simulink library "M160_lib"  (Simulink 7.8)
settings: Solver=FixedStepDiscrete  StartTime=0.0  StopTime=10.0  RelTol=1e-3
PreLoadFcn:
  | update_path
undefined symbols (not defined in the file): Afr_atCool2facLambdaReqCorr_CUR_x, Afr_atCool2facLambdaReqCorr_CUR_y, Afr_atMani2facLambdaReqCorr_CUR_x, Afr_atMani2facLambdaReqCorr_CUR_y, Afr_facLambdaReqMan, Afr_facRatioMan, Afr_facStoich, Afr_flgLambdaReqOverride, Afr_flgRatioOverride, Afr_rpmEngSpdfacRelAir2facLambdaReqBase_MAP_x, Afr_rpmEngSpdfacRelAir2facLambdaReqBase_MAP_y, Afr_rpmEngSpdfacRelAir2facLambdaReqBase_MAP_z, Ais_flgAirInjReacPumpOverride, Ais_stAirInjReacPumpMan, Amc_flgAirMassFlowOverride, Amc_uSens2AirMassFlow_CUR_x, Amc_uSens2AirMassFlow_CUR_y, Amc_uSensMaxValid, Amc_uSensMinValid, Amf_facRelAirMan, Amf_flgAirMassPerStrOverride, Amf_flgRelAirOverride, Amf_flgSwitch2AirMassFlowMeter, Amf_mAirPerStrMan, Amf_pManiEngSpd2facRelAirCorr_MAP_x, Amf_pManiEngSpd2facRelAirCorr_MAP_y, Amf_pManiEngSpd2facRelAirCorr_MAP_z, Amf_rpmEngSpd2facTempCorr_CUR_x, Amf_rpmEngSpd2facTempCorr_CUR_y, Amf_shcSpecGasConst_C, Amf_volEngDisp_C, Apv_facAirPumpRateMan, Apv_factor, Apv_flgAirPumpRateOverride, Apv_tiPeriod_C, Bvc_rVoltDivHigh, Bvc_rVoltDivLow, Bvc_uBattMax, Bvc_uBattMin, CDRV_E_OK_, Cov_facChOverVlvRateMan, Cov_factor, Cov_flgChOverVlvRateOverride, Cov_tiPeriod_C, Cpc_atManiTmp2facPresCorr_CUR_x, Cpc_atManiTmp2facPresCorr_CUR_y, Cpc_flgPChargeOverride, Cpc_uSens2pManiBase_CUR_x, Cpc_uSens2pManiBase_CUR_y, Ctc_rPullUp_C, Ctc_rSens2atCool_CUR_x, Ctc_rSens2atCool_CUR_y, Ctc_uSensMaxValid, Ctc_uSensMinValid, Ctc_uSupply, Doh_OutputDiagnosisOverride, dummy_facAirPumpRateReq, dummy_facChOverVlvRateReq, dummy_flgInterCoolerOverride, dummy_flgKl50Override ... (+243)
libraries: simulink x36, ehooks_lib x3
(part 1 of 8)
CloseFcn:
  | clear
settings Model: Creator=WLB9FE  LastModifiedBy=Tiger

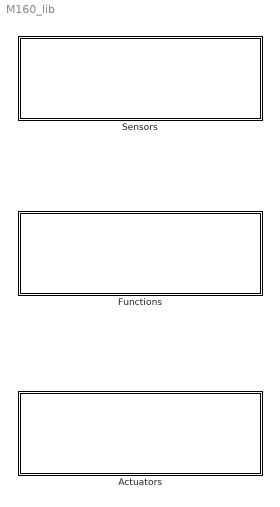
== system M160_lib ==
  Actuators : Subsystem
      mask Display: fprintf('actuators')
  Functions : Subsystem
      mask Display: fprintf('functions')
  Sensors : Subsystem
      mask Display: fprintf('sensors')

== system M160_lib/Actuators ==
  Ais : Subsystem
      mask Type: Actuators
      mask Description: AirInjectionReactorPump
      mask Display:
      | image(imread('AirInjectionReactorPump.jpg'))
      | port_label('input',1,'Opm_idxMode')
      | port_label('input',2,'dummy_stAirInjReacPump')
      | port_label('output',1,'Ais_stDiagnosis')
      | port_label('output',2,'Ais_flgError')
  Apv : Subsystem
      mask Type: Actuators
      mask Description: AirPumpValve
      mask Display:
      | image(imread('AirPumpValve.jpg'))
      | port_label('input',1,'Opm_idxMode')
      | port_label('input',2,'dummy_facAirPumpRate')
      | port_label('output',1,'Apv_stDiagnosis')
      | port_label('output',2,'Apv_flgError')
  Cov : Subsystem
      mask Type: Actuators
      mask Description: ChangeOverValve
      mask Display:
      | image(imread('ChangeOverValve.jpg'))
      | port_label('input',1,'Opm_idxMode')
      | port_label('input',2,'dummy_facChOverVlvRate')
      | port_label('output',1,'Cov_stDiagnosis')
      | port_label('output',2,'Cov_flgError')
  Fps : Subsystem
      mask Type: Actuators
      mask Description: FuelPump
      mask Display:
      | image(imread('FuelPump.jpg'))
      | port_label('input',1,'Opm_idxMode')
      | port_label('input',2,'dummy_stFuelPump')
      | port_label('output',1,'Fps_stDiagnosis')
      | port_label('output',2,'Fps_flgError')
  Icc : Subsystem
      mask Type: Actuators
      mask Description: IgnitionCoil
      mask Display:
      | image(imread('IgnitionCoil.jpg'))
      | port_label('input',1,'Opm_idxMode')
      | port_label('input',2,'Iac_flgIgnCutoff')
      | port_label('input',3,'Iac_degIgnIdleSpeed')
      | port_label('output',1,'Icc_flgError')
  Ics : Subsystem
      mask Type: Actuators
      mask Description: Intercooler
      mask Display:
      | image(imread('Intercooler.jpg'))
      | port_label('input',1,'Opm_idxMode')
      | port_label('input',2,'dummy_stIntercooler')
      | port_label('output',1,'Ics_stDiagnosis')
      | port_label('output',2,'Ics_flgError')
  Ivc : Subsystem
      mask Type: Actuators
      mask Description: InjectionValve
      mask Display:
      | image(imread('InjectionValve.jpg'))
      | port_label('input',1,'Opm_idxMode')
      | port_label('input',2,'Itc_flgInjCutoff')
      | port_label('input',3,'Itc_tiInj')
      | port_label('input',4,'Itc_tiBattDelay')
      | port_label('output',1,'Ivc_flgError')
  Mrs : Subsystem
      mask Type: Actuators
      mask Description: MainRelais
      mask Display:
      | image(imread('MainRelais.jpg'))
      | port_label('input',1,'Opm_idxMode')
      | port_label('input',2,'dummy_stMainRelais')
      | port_label('output',1,'Mrs_stDiagnosis')
      | port_label('output',2,'Mrs_flgError')
  Str : Subsystem
      mask Type: Actuators
      mask Description: Starter
      mask Display:
      | image(imread('Starter.jpg'))
      | port_label('input',1,'Opm_idxMode')
      | port_label('input',2,'Stc_stStarter')
      | port_label('output',1,'Str_stDiagnosis')
      | port_label('output',2,'Str_flgError')
  Tvc : Subsystem
      mask Type: Actuators
      mask Description: ThrottleValve
      mask Display:
      | image(imread('ThrottleValve.jpg'))
      | port_label('input',1,'Opm_idxMode')
      | port_label('input',2,'dummy_facThrValveReq')
      | port_label('output',1,'Tvc_stDiagnosis')
      | port_label('output',2,'Tvc_flgError')
  Wcs : Subsystem
      mask Type: Actuators
      mask Description: WaterCooler
      mask Display:
      | image(imread('WaterCooler.jpg'))
      | port_label('input',1,'Opm_idxMode')
      | port_label('input',2,'Ctc_atCool')
      | port_label('output',1,'Wcs_stDiagnosis')
      | port_label('output',2,'Wcs_flgError')
  Wgc : Subsystem
      mask Type: Actuators
      mask Description: WasteGate
      mask Display:
      | image(imread('WasteGate.jpg'))
      | port_label('input',1,'Opm_idxMode')
      | port_label('input',2,'T2t_facWasteGateRate')
      | port_label('output',1,'Wgc_stDiagnosis')
      | port_label('output',2,'Wgc_flgError')

== system M160_lib/Functions ==
  Afr : Subsystem
      mask Type: Functions
      mask Description: AirFuelRatio
      mask Display:
      | image(imread('AirFuelRatio.jpg'))
      | port_label('input',1,'Epm_rpmEngSpd')
      | port_label('input',2,'Mtc_atMani')
      | port_label('input',3,'Ctc_atCool')
      | port_label('input',4,'Amf_facRelAir')
      | port_label('output',1,'Afr_facLambdaReq')
      | port_label('output',2,'Afr_facRatio')
  Amf : Subsystem
      mask Type: Functions
      mask Description: AirMassFlow
      mask Display:
      | image(imread('AirMassFlow.jpg'))
      | port_label('input',1,'Epm_rpmEngSpd')
      | port_label('input',2,'Mtc_atMani')
      | port_label('input',3,'Mpc_pManiFilt')
      | port_label('input',4,'Ctc_atCool')
      | port_label('input',5,'Amc_AirMassFlow')
      | port_label('output',1,'Amf_mAirPerStr')
      | port_label('output',2,'Amf_facRelAir')
  Doh : Subsystem
      mask Type: Functions
      mask Description: DiagnosisOutput
      mask Display:
      | image(imread('DiagnosisOutput.jpg'))
      | port_label('input',1,'Tvc_stDiagnosis')
      | port_label('input',2,'Mrs_stDiagnosis')
      | port_label('input',3,'Fps_stDiagnosis')
      | port_label('input',4,'Wcs_stDiagnosis')
      | port_label('input',5,'Wgc_stDiagnosis')
      | port_label('input',6,'Ics_stDiagnosis')
      | port_label('input',7,'Apv_stDiagnosis')
      | port_label('input',8,'Ais_stDiagnosis')
      | port_label('input',9,'Cov_stDiagnosis')
      | port_label('input',10,'Str_stDiagnosis')
      | port_label('output',1,'Doh_flgErrorDiagnosis')
  Dummy : Subsystem
      mask Type: Functions
      mask Description: Dummy
      mask Display:
      | image(imread('Dummy.jpg'))
      | port_label('input',1,'T2t_facThrValveReq')
      | port_label('input',2,'Egc_facEgas')
      | port_label('input',3,'Epm_rpmEngSpd')
      | port_label('input',4,'ICC_flgInterCooler')
      | port_label('input',5,'Kl50_stKlemme50')
      | port_label('output',1,'dummy_facThrValveReq')
      | port_label('output',2,'dummy_facAirPumpRate')
      | port_label('output',3,'dummy_facChOverVlvRate')
      | port_label('output',4,'dummy_stMainRelais')
      | port_label('output',5,'dummy_stFuelPump')
      | port_label('output',6,'dummy_stIntercooler')
      | port_label('output',7,'dummy_stAirInjReacPump')
      | port_label('output',8,'dummy_Starter')
  Eih : Subsystem
      mask Type: Functions
      mask Description: ErrorInput
      mask Display:
      | image(imread('ErrorInput.jpg'))
      | port_label('input',1,'Egc_flgError')
      | port_label('input',2,'Ctc_flgError')
      | port_label('input',3,'Mtc_flgError')
      | port_label('input',4,'Mpc_flgError')
      | port_label('input',5,'Cpc_flgError')
      | port_label('input',6,'Bvc_flgError')
      | port_label('input',7,'Opc_flgError')
      | port_label('input',8,'Amc_flgError')
      | port_label('input',9,'Kl50_flgError')
      | port_label('output',1,'Eih_flgInputError')
  Eoh : Subsystem
      mask Type: Functions
      mask Description: ErrorOutput
      mask Display:
      | image(imread('ErrorOutput.jpg'))
      | port_label('input',1,'Tvc_flgError')
      | port_label('input',2,'Mrs_flgError')
      | port_label('input',3,'Icc_flgError')
      | port_label('input',4,'Fps_flgError')
      | port_label('input',5,'Ivc_flgError')
      | port_label('input',6,'Wcs_flgError')
      | port_label('input',7,'Wgc_flgError')
      | port_label('input',8,'Ics_flgError')
      | port_label('input',9,'Apv_flgError')
      | port_label('input',10,'Ais_flgError')
      | port_label('input',11,'Cov_flgError')
      | port_label('input',12,'Str_flgError')
      | port_label('output',1,'Eih_flgInputError')
  Fmc : Subsystem
      mask Type: Functions
      mask Description: FuelMass
      mask Display:
      | image(imread('FuelMass.jpg'))
      | port_label('input',1,'Epm_rpmEngSpd')
      | port_label('input',2,'Lcc_facLambdaCorr')
      | port_label('input',3,'Afr_facRatio')
      | port_label('input',4,'Amf_mAirPerStr')
      | port_label('input',5,'Tqs_tqReq')
      | port_label('input',6,'Itc_tiInjOffset')
      | port_label('output',1,'Fmc_mFuel')
  ICC_1 : Subsystem
      mask Type: Functions
      mask Description: InterCoolerControl
      mask Display:
      | image(imread('InterCoolerControl.jpg'))
      | port_label('input',1,'Mpc_pManiFilt')
      | port_label('output',1,'ICC_flgInterCooler')
  Iac : Subsystem
      mask Type: Functions
      mask Description: IgnitionAngle
      mask Display:
      | image(imread('IgnitionAngle.jpg'))
      | port_label('input',1,'Epm_rpmEngSpd')
      | port_label('input',2,'Amf_facRelAir')
      | port_label('input',3,'Mpc_pManiFilt')
      | port_label('input',4,'Isc_flgIdleSpdCtrlActive')
      | port_label('input',5,'T2t_pManiReqFast')
      | port_label('input',6,'Stc_flgCatalyserHeating')
      | port_label('output',1,'Iac_flgIgnCutoff')
      | port_label('output',2,'Iac_degIgnIdleSpeed')
      | port_label('output',3,'Iac_degIgn')
      | port_label('output',4,'Iac_degMinAdvBestTq')
  Isc : Subsystem
      mask Type: Functions
      mask Description: IdleSpeedController
      mask Display:
      | image(imread('IdleSpeedController.jpg'))
      | port_label('input',1,'Epm_rpmEngSpd')
      | port_label('input',2,'Egc_facEgas')
      | port_label('input',3,'Stc_flgStarterActive')
      | port_label('input',4,'Stc_flgCatalyserHeating')
      | port_label('input',5,'Stc_CatalyserHeatingTime')
      | port_label('output',1,'Isc_flgFuelCutoff')
      | port_label('output',2,'Isc_facIdleSpdStab')
      | port_label('output',3,'Isc_IdleSpdCtrlIPart')
      | port_label('output',4,'Isc_IdleSpdCtrlPPart')
      | port_label('output',5,'Isc_flgIdleSpdCtrlActive')
  Itc : Subsystem
      mask Type: Functions
      mask Description: InjectionTime
      mask Display:
      | image(imread('InjectionTime.jpg'))
      | port_label('input',1,'Epm_rpmEngSpd')
      | port_label('input',2,'Bvc_uBatt')
      | port_label('input',3,'Mpc_pManiFilt')
      | port_label('input',4,'Isc_flgFuelCutoff')
      | port_label('input',5,'Fmc_mFuel')
      | port_label('input',6,'Iac_flgIgnCutoff')
      | port_label('input',7,'Stc_facFuelCorr')
      | port_label('output',1,'Itc_flgInjCutoff')
      | port_label('output',2,'Itc_tiInj')
      | port_label('output',3,'Itc_tiBattDelay')
      | port_label('output',4,'Itc_tiInjOffset')
  Lcc : Subsystem
      mask Type: Functions
      mask Description: LambdaControl
      mask Display:
      | image(imread('LambdaControl.jpg'))
      | port_label('input',1,'Epm_rpmEngSpd')
      | port_label('input',2,'Isc_flgFuelCutoff')
      | port_label('input',3,'Lamsoni')
      | port_label('input',4,'Afr_facLambdaReq')
      | port_label('input',5,'Stc_flgFuelCorrActive')
      | port_label('input',6,'Mpc_pManiFilt')
      | port_label('output',1,'Lcc_facLambdaCorr')
  Opm : Subsystem
      mask Type: Functions
      mask Description: OperationMode
      mask Display:
      | image(imread('OperationMode.jpg'))
      | port_label('input',1,'Eih_flgInputError')
      | port_label('input',2,'Doh_flgErrorDiagnosis')
      | port_label('input',3,'Eoh_flgOutputError')
      | port_label('output',1,'Opm_idxMode')
  Stc : Subsystem
      mask Type: Functions
      mask Description: StarterControl
      mask Display:
      | image(imread('StarterControl.jpg'))
      | port_label('input',1,'Epm_rpmEngSpd')
      | port_label('input',2,'dummy_Starter')
      | port_label('input',3,'Opm_idxMode')
      | port_label('input',4,'Ctc_atCool')
      | port_label('output',1,'Stc_flgFuelCorrActive')
      | port_label('output',2,'Stc_flgStarterActive')
      | port_label('output',3,'Stc_CatalyserHeatingTime')
      | port_label('output',4,'Stc_facFuelCorr')
      | port_label('output',5,'Stc_stStarter')
      | port_label('output',6,'Stc_flgCatalyserHeating')
  T2t : Subsystem
      mask Type: Functions
      mask Description: Torque2Throttle
      mask Display:
      | image(imread('Torque2Throttle.jpg'))
      | port_label('input',1,'Epm_rpmEngSpd')
      | port_label('input',2,'Iac_degIgn')
      | port_label('input',3,'Iac_degMinAdvBestTq')
      | port_label('input',4,'Afr_facLambdaReq')
      | port_label('input',5,'Tqs_tqReq')
      | port_label('input',6,'Mpc_pManiFilt')
      | port_label('input',7,'Isc_IdleSpdCtrlIPart')
      | port_label('input',8,'Isc_IdleSpdCtrlPPart')
      | port_label('input',9,'Isc_flgIdleSpdCtrlActive')
      | port_label('input',10,'Stc_flgStarterActive')
      | port_label('input',11,'Stc_flgCatalyserHeating')
      | port_label('input',12,'Stc_CatalyserHeatingTime')
      | port_label('output',1,'T2t_pManiReqFast')
      | port_label('output',2,'T2t_facWasteGateRate')
      | port_label('output',3,'T2t_facThrValveReq')
  Tqs : Subsystem
      mask Type: Functions
      mask Description: TorqueStructure
      mask Display:
      | image(imread('TorqueStructure.jpg'))
      | port_label('input',1,'Epm_rpmEngSpd')
      | port_label('input',2,'Amf_facRelAir')
      | port_label('input',3,'Ctc_atCool')
      | port_label('input',4,'Egc_facEgas')
      | port_label('input',5,'Isc_facIdleSpdStab')
      | port_label('output',1,'Tqs_tqReq')

== system M160_lib/Sensors ==
  Amc : Subsystem
      mask Type: Sensors
      mask Description: AirMassFlowMeter
      mask Display:
      | image(imread('AirMassFlowMeter.jpg'))
      | port_label('output',1,'Amc_flgError')
      | port_label('output',2,'Amc_AirMassFlow')
  Bvc : Subsystem
      mask Type: Sensors
      mask Description: BatteryVoltage
      mask Display:
      | image(imread('BatteryVoltage.jpg'))
      | port_label('output',1,'Bvc_flgError')
      | port_label('output',2,'Bvc_uBatt')
  Cpc : Subsystem
      mask Type: Sensors
      mask Description: ChargingPressure
      mask Display:
      | image(imread('ChargingPressure.jpg'))
      | port_label('input',1,'Epm_rpmEngSpd')
      | port_label('input',2,'Mtc_atMani')
      | port_label('output',1,'Cpc_flgError')
      | port_label('output',2,'Cpc_pchargeFilt')
  Ctc : Subsystem
      mask Type: Sensors
      mask Description: CoolantTemperature
      mask Display:
      | image(imread('CoolantTemperature.jpg'))
      | port_label('output',1,'Ctc_flgError')
      | port_label('output',2,'Ctc_atCool')
  Egc : Subsystem
      mask Type: Sensors
      mask Description: Egas
      mask Display:
      | image(imread('Egas.jpg'))
      | port_label('output',1,'Egc_flgError')
      | port_label('output',2,'Egc_facEgas')
  Klemme50 : Subsystem
      mask Type: Sensors
      mask Description: Klemme50
      mask Display:
      | image(imread('Klemme50.jpg'))
      | port_label('output',1,'Kl50_flgError')
      | port_label('output',2,'Kl50_stKlemme50')
  Mpc : Subsystem
      mask Type: Sensors
      mask Description: ManifoldPressure
      mask Display:
      | image(imread('ManifoldPressure.jpg'))
      | port_label('input',1,'Epm_rpmEngSpd')
      | port_label('input',2,'Mtc_atMani')
      | port_label('output',1,'Mpc_flgError')
      | port_label('output',2,'Mpc_pManiFilt')
  Mtc : Subsystem
      mask Type: Sensors
      mask Description: ManifoldTemperature
      mask Display:
      | image(imread('ManifoldTemperature.jpg'))
      | port_label('output',1,'Mtc_flgError')
      | port_label('output',2,'Mtc_atManil')
  Opc : Subsystem
      mask Type: Sensors
      mask Description: OilPressure
      mask Display:
      | image(imread('OilPressure.jpg'))
      | port_label('input',1,'Epm_rpmEngSpd')
      | port_label('output',1,'Opc_flgError')
      | port_label('output',2,'Opc_stOilPressure')

== system M160_lib/Actuators/Ais ==
  Opm_idxMode : Inport
  dummy_stAirInjReacPump : Inport  Port=2
  function : TriggerPort  TriggerType=function-call
  Constant1 : Constant  Value=Ais_flgAirInjReacPumpOverride
  Constant2 : Constant  Value=Ais_stAirInjReacPumpMan
  Constant5 : Constant  Value=Normal
  Constant6 : Constant  Value=0  OutDataTypeStr=boolean
  G1_DigOut_Ctrl : Subsystem  AncestorBlock=ehooks_medc17flex_G1_lib/Library Blocks/Basic_IO/Outputs/G1_DigOut_Ctrl  LoadFcn=ehooks_medc17flex_devlib_io_block('load');  InitFcn=ehooks_medc17flex_devlib_io_block('init');  StartFcn=ehooks_medc17flex_devlib_io_block('start');  StopFcn=ehooks_medc17flex_devlib_io_block('stop');  ClipboardFcn=ehooks_medc17flex_devlib_io_block('clipboard', 0); % Second argument just needed to indicate null block. See callback handler.  mask{ChannelName=O_S_RL30}
      mask prompts: ChannelName "Channel name"
      mask init:
      | ehooks_medc17flex_devlib_io_block('mask_init');
      settings: AttributesFormatString=Channel name: '%<ChannelName>'  CopyFcn=ehooks_medc17flex_devlib_io_block('copy');  DeleteFcn=ehooks_medc17flex_devlib_io_block('delete');  UndoDeleteFcn=ehooks_medc17flex_devlib_io_block('undo_delete');  ModelCloseFcn=ehooks_medc17flex_devlib_io_block('model_close');  PreSaveFcn=ehooks_medc17flex_devlib_io_block('pre_save');  PostSaveFcn=ehooks_medc17flex_devlib_io_block('post_save');  NameChangeFcn=ehooks_medc17flex_devlib_io_block('name_change');  DestroyFcn=ehooks_medc17flex_devlib_io_block('destroy', 0); % Second argument just needed to indicate null block. See callback handler.  OpenFcn=ehooks_medc17flex_devlib_io_block('open');  CloseFcn=ehooks_medc17flex_devlib_io_block('close');  ParentCloseFcn=ehooks_medc17flex_devlib_io_block('parent_close');  MoveFcn=ehooks_medc17flex_devlib_io_block('move');
      mask StyleString: popup(<empty>|O_S_MRLY|O_S_RL09|O_S_RL14|O_S_RL29|O_S_RL30|O_S_RL31|O_S_RL33|O_S_RL34|O_S_RL35|O_S_RL41|O_S_RL43)
      mask Display: image(imread('Output_Digital.jpg'))
  G1_DigOut_GetError : Subsystem  AncestorBlock=ehooks_medc17flex_G1_lib/Library Blocks/Basic_IO/Outputs/G1_DigOut_GetError  LoadFcn=ehooks_medc17flex_devlib_io_block('load');  InitFcn=ehooks_medc17flex_devlib_io_block('init');  StartFcn=ehooks_medc17flex_devlib_io_block('start');  StopFcn=ehooks_medc17flex_devlib_io_block('stop');  ClipboardFcn=ehooks_medc17flex_devlib_io_block('clipboard', 0); % Second argument just needed to indicate null block. See callback handler.  mask{ChannelName=O_S_RL30}
      mask prompts: ChannelName "Channel name"
      mask init:
      | ehooks_medc17flex_devlib_io_block('mask_init');
      settings: AttributesFormatString=Channel name: '%<ChannelName>'  CopyFcn=ehooks_medc17flex_devlib_io_block('copy');  DeleteFcn=ehooks_medc17flex_devlib_io_block('delete');  UndoDeleteFcn=ehooks_medc17flex_devlib_io_block('undo_delete');  ModelCloseFcn=ehooks_medc17flex_devlib_io_block('model_close');  PreSaveFcn=ehooks_medc17flex_devlib_io_block('pre_save');  PostSaveFcn=ehooks_medc17flex_devlib_io_block('post_save');  NameChangeFcn=ehooks_medc17flex_devlib_io_block('name_change');  DestroyFcn=ehooks_medc17flex_devlib_io_block('destroy', 0); % Second argument just needed to indicate null block. See callback handler.  OpenFcn=ehooks_medc17flex_devlib_io_block('open');  CloseFcn=ehooks_medc17flex_devlib_io_block('close');  ParentCloseFcn=ehooks_medc17flex_devlib_io_block('parent_close');  MoveFcn=ehooks_medc17flex_devlib_io_block('move');
      mask StyleString: popup(<empty>|O_S_MRLY|O_S_RL09|O_S_RL14|O_S_RL29|O_S_RL30|O_S_RL31|O_S_RL33|O_S_RL34|O_S_RL35|O_S_RL41|O_S_RL43)
      mask Display: image(imread('Output_Digital_Diagnosis.jpg'))
  Logical Operator1 : Logic  Operator=NOT  AllPortsSameDT=off  OutDataTypeStr=boolean
  Logical Operator2 : Logic  Operator=NOT  AllPortsSameDT=off  OutDataTypeStr=boolean
  Relational Operator : RelationalOperator  Operator===  OutDataTypeStr=boolean
  Switch1 : Switch  Threshold=1
  Switch2 : Switch  Threshold=1
  Ais_stDiagnosis : Outport
  Ais_flgError : Outport  Port=2
  wires:
  G1_DigOut_Ctrl/1(status) -> Logical Operator1/1
  Logical Operator2/1 -> G1_DigOut_Ctrl/1(state)
  Switch2/1 -> Logical Operator2/1  "Ais_stAirInjReacPump"
  G1_DigOut_GetError/1(status) -> Ais_stDiagnosis/1  "Ais_stDiagnosis"
  Logical Operator1/1 -> Ais_flgError/1  "Ais_flgError"
  Constant1/1 -> Switch1/2
  Constant2/1 -> Switch1/1
  dummy_stAirInjReacPump/1 -> Switch1/3
  Switch1/1 -> Switch2/1
  Opm_idxMode/1 -> Relational Operator/1
  Constant5/1 -> Relational Operator/2
  Relational Operator/1 -> Switch2/2
  Constant6/1 -> Switch2/3

== system M160_lib/Actuators/Apv ==
  Opm_idxMode : Inport
  dummy_facAirPumpRate : Inport  Port=2
  function : TriggerPort  TriggerType=function-call
  Constant1 : Constant  Value=Apv_flgAirPumpRateOverride
  Constant2 : Constant  Value=Apv_facAirPumpRateMan
  Constant3 : Constant  Value=10000  OutDataTypeStr=single
  Constant4 : Constant  Value=Apv_factor
  Constant5 : Constant  Value=Normal
  Constant6 : Constant  Value=0.05  OutDataTypeStr=single
  Constant7 : Constant  Value=Apv_tiPeriod_C
  Constant9 : Constant  Value=Lo_
  G1_PWM_Output_Ctrl : Subsystem  AncestorBlock=ehooks_medc17flex_G1_lib/Library Blocks/Basic_IO/Outputs/G1_PWM_Output_Ctrl  LoadFcn=ehooks_medc17flex_devlib_io_block('load');  InitFcn=ehooks_medc17flex_devlib_io_block('init');  StartFcn=ehooks_medc17flex_devlib_io_block('start');  StopFcn=ehooks_medc17flex_devlib_io_block('stop');  ClipboardFcn=ehooks_medc17flex_devlib_io_block('clipboard', 0); % Second argument just needed to indicate null block. See callback handler.  mask{ChannelName=O_T_RL13}
      mask prompts: ChannelName "Channel name"
      mask init:
      | ehooks_medc17flex_devlib_io_block('mask_init');
      settings: AttributesFormatString=Channel name: '%<ChannelName>'  CopyFcn=ehooks_medc17flex_devlib_io_block('copy');  DeleteFcn=ehooks_medc17flex_devlib_io_block('delete');  UndoDeleteFcn=ehooks_medc17flex_devlib_io_block('undo_delete');  ModelCloseFcn=ehooks_medc17flex_devlib_io_block('model_close');  PreSaveFcn=ehooks_medc17flex_devlib_io_block('pre_save');  PostSaveFcn=ehooks_medc17flex_devlib_io_block('post_save');  NameChangeFcn=ehooks_medc17flex_devlib_io_block('name_change');  DestroyFcn=ehooks_medc17flex_devlib_io_block('destroy', 0); % Second argument just needed to indicate null block. See callback handler.  OpenFcn=ehooks_medc17flex_devlib_io_block('open');  CloseFcn=ehooks_medc17flex_devlib_io_block('close');  ParentCloseFcn=ehooks_medc17flex_devlib_io_block('parent_close');  MoveFcn=ehooks_medc17flex_devlib_io_block('move');
      mask StyleString: popup(<empty>|O_T_RL10|O_T_RL13|O_T_RL19|O_T_RL20|O_T_RL22|O_T_RL23|O_T_RL25|O_T_RL26|O_T_RL27|O_T_RL28|O_T_RL38|O_T_RL39|O_T_RL40|O_T_RL42|O_T_RL44|O_T_RL45|O_T_RL46|O_T_RL47|O_T_RL48|O_T_RL49|O_T_RL50|O_T_RH02)
      mask Display: image(imread('Output_PWM.jpg'))
  G1_PwmOut_Get_error : Subsystem  AncestorBlock=ehooks_medc17flex_G1_lib/Library Blocks/Basic_IO/Outputs/G1_PwmOut_Get_error  LoadFcn=ehooks_medc17flex_devlib_io_block('load');  InitFcn=ehooks_medc17flex_devlib_io_block('init');  StartFcn=ehooks_medc17flex_devlib_io_block('start');  StopFcn=ehooks_medc17flex_devlib_io_block('stop');  ClipboardFcn=ehooks_medc17flex_devlib_io_block('clipboard', 0); % Second argument just needed to indicate null block. See callback handler.  mask{ChannelName=O_T_RL13}
      mask prompts: ChannelName "Channel name"
      mask init:
      | ehooks_medc17flex_devlib_io_block('mask_init');
      settings: AttributesFormatString=Channel name: '%<ChannelName>'  CopyFcn=ehooks_medc17flex_devlib_io_block('copy');  DeleteFcn=ehooks_medc17flex_devlib_io_block('delete');  UndoDeleteFcn=ehooks_medc17flex_devlib_io_block('undo_delete');  ModelCloseFcn=ehooks_medc17flex_devlib_io_block('model_close');  PreSaveFcn=ehooks_medc17flex_devlib_io_block('pre_save');  PostSaveFcn=ehooks_medc17flex_devlib_io_block('post_save');  NameChangeFcn=ehooks_medc17flex_devlib_io_block('name_change');  DestroyFcn=ehooks_medc17flex_devlib_io_block('destroy', 0); % Second argument just needed to indicate null block. See callback handler.  OpenFcn=ehooks_medc17flex_devlib_io_block('open');  CloseFcn=ehooks_medc17flex_devlib_io_block('close');  ParentCloseFcn=ehooks_medc17flex_devlib_io_block('parent_close');  MoveFcn=ehooks_medc17flex_devlib_io_block('move');
      mask StyleString: popup(<empty>|O_T_RL10|O_T_RL13|O_T_RL19|O_T_RL20|O_T_RL22|O_T_RL23|O_T_RL25|O_T_RL26|O_T_RL27|O_T_RL28|O_T_RL38|O_T_RL39|O_T_RL40|O_T_RL42|O_T_RL44|O_T_RL45|O_T_RL46|O_T_RL47|O_T_RL48|O_T_RL49|O_T_RL50|O_T_RH02)
      mask Display: image(imread('Output_PWM_Diagnosis.jpg'))
  Logical Operator1 : Logic  Operator=NOT  AllPortsSameDT=off  OutDataTypeStr=boolean
  Product1 : Product  OutDataTypeStr=Inherit: Same as first input
  Relational Operator : RelationalOperator  Operator===  OutDataTypeStr=boolean
  Switch1 : Switch  Threshold=1
  Switch2 : Switch  Threshold=1
  Apv_stDiagnosis : Outport
  Apv_flgError : Outport  Port=2
  wires:
  Constant9/1 -> G1_PWM_Output_Ctrl/4(level)
  Constant4/1 -> G1_PWM_Output_Ctrl/3(factor)
  Constant7/1 -> G1_PWM_Output_Ctrl/2(period)
  Product1/1 -> G1_PWM_Output_Ctrl/1(dutycycle)
  Constant3/1 -> Product1/2
  G1_PWM_Output_Ctrl/1(status) -> Logical Operator1/1
  Switch2/1 -> Product1/1  "Apv_facAirPumpRate"
  G1_PwmOut_Get_error/1(status) -> Apv_stDiagnosis/1  "Apv_stDiagnosis"
  Logical Operator1/1 -> Apv_flgError/1  "Apv_flgError"
  Constant1/1 -> Switch1/2
  Constant2/1 -> Switch1/1
  dummy_facAirPumpRate/1 -> Switch1/3
  Switch1/1 -> Switch2/1
  Opm_idxMode/1 -> Relational Operator/1
  Constant5/1 -> Relational Operator/2
  Relational Operator/1 -> Switch2/2
  Constant6/1 -> Switch2/3

== system M160_lib/Actuators/Cov ==
  Opm_idxMode : Inport
  dummy_facChOverVlvRate : Inport  Port=2
  function : TriggerPort  TriggerType=function-call
  Constant1 : Constant  Value=Cov_flgChOverVlvRateOverride
  Constant2 : Constant  Value=Cov_facChOverVlvRateMan
  Constant3 : Constant  Value=10000  OutDataTypeStr=single
  Constant4 : Constant  Value=Cov_factor
  Constant5 : Constant  Value=Normal
  Constant6 : Constant  Value=0.05  OutDataTypeStr=single
  Constant7 : Constant  Value=Cov_tiPeriod_C
  Constant9 : Constant  Value=Lo_
  G1_PWM_Output_Ctrl : Subsystem  AncestorBlock=ehooks_medc17flex_G1_lib/Library Blocks/Basic_IO/Outputs/G1_PWM_Output_Ctrl  LoadFcn=ehooks_medc17flex_devlib_io_block('load');  InitFcn=ehooks_medc17flex_devlib_io_block('init');  StartFcn=ehooks_medc17flex_devlib_io_block('start');  StopFcn=ehooks_medc17flex_devlib_io_block('stop');  ClipboardFcn=ehooks_medc17flex_devlib_io_block('clipboard', 0); % Second argument just needed to indicate null block. See callback handler.  mask{ChannelName=O_T_RL10}
      mask prompts: ChannelName "Channel name"
      mask init:
      | ehooks_medc17flex_devlib_io_block('mask_init');
      settings: AttributesFormatString=Channel name: '%<ChannelName>'  CopyFcn=ehooks_medc17flex_devlib_io_block('copy');  DeleteFcn=ehooks_medc17flex_devlib_io_block('delete');  UndoDeleteFcn=ehooks_medc17flex_devlib_io_block('undo_delete');  ModelCloseFcn=ehooks_medc17flex_devlib_io_block('model_close');  PreSaveFcn=ehooks_medc17flex_devlib_io_block('pre_save');  PostSaveFcn=ehooks_medc17flex_devlib_io_block('post_save');  NameChangeFcn=ehooks_medc17flex_devlib_io_block('name_change');  DestroyFcn=ehooks_medc17flex_devlib_io_block('destroy', 0); % Second argument just needed to indicate null block. See callback handler.  OpenFcn=ehooks_medc17flex_devlib_io_block('open');  CloseFcn=ehooks_medc17flex_devlib_io_block('close');  ParentCloseFcn=ehooks_medc17flex_devlib_io_block('parent_close');  MoveFcn=ehooks_medc17flex_devlib_io_block('move');
      mask StyleString: popup(<empty>|O_T_RL10|O_T_RL13|O_T_RL19|O_T_RL20|O_T_RL22|O_T_RL23|O_T_RL25|O_T_RL26|O_T_RL27|O_T_RL28|O_T_RL38|O_T_RL39|O_T_RL40|O_T_RL42|O_T_RL44|O_T_RL45|O_T_RL46|O_T_RL47|O_T_RL48|O_T_RL49|O_T_RL50|O_T_RH02)
      mask Display: image(imread('Output_PWM.jpg'))
  G1_PwmOut_Get_error : Subsystem  AncestorBlock=ehooks_medc17flex_G1_lib/Library Blocks/Basic_IO/Outputs/G1_PwmOut_Get_error  LoadFcn=ehooks_medc17flex_devlib_io_block('load');  InitFcn=ehooks_medc17flex_devlib_io_block('init');  StartFcn=ehooks_medc17flex_devlib_io_block('start');  StopFcn=ehooks_medc17flex_devlib_io_block('stop');  ClipboardFcn=ehooks_medc17flex_devlib_io_block('clipboard', 0); % Second argument just needed to indicate null block. See callback handler.  mask{ChannelName=O_T_RL10}
      mask prompts: ChannelName "Channel name"
      mask init:
      | ehooks_medc17flex_devlib_io_block('mask_init');
      settings: AttributesFormatString=Channel name: '%<ChannelName>'  CopyFcn=ehooks_medc17flex_devlib_io_block('copy');  DeleteFcn=ehooks_medc17flex_devlib_io_block('delete');  UndoDeleteFcn=ehooks_medc17flex_devlib_io_block('undo_delete');  ModelCloseFcn=ehooks_medc17flex_devlib_io_block('model_close');  PreSaveFcn=ehooks_medc17flex_devlib_io_block('pre_save');  PostSaveFcn=ehooks_medc17flex_devlib_io_block('post_save');  NameChangeFcn=ehooks_medc17flex_devlib_io_block('name_change');  DestroyFcn=ehooks_medc17flex_devlib_io_block('destroy', 0); % Second argument just needed to indicate null block. See callback handler.  OpenFcn=ehooks_medc17flex_devlib_io_block('open');  CloseFcn=ehooks_medc17flex_devlib_io_block('close');  ParentCloseFcn=ehooks_medc17flex_devlib_io_block('parent_close');  MoveFcn=ehooks_medc17flex_devlib_io_block('move');
      mask StyleString: popup(<empty>|O_T_RL10|O_T_RL13|O_T_RL19|O_T_RL20|O_T_RL22|O_T_RL23|O_T_RL25|O_T_RL26|O_T_RL27|O_T_RL28|O_T_RL38|O_T_RL39|O_T_RL40|O_T_RL42|O_T_RL44|O_T_RL45|O_T_RL46|O_T_RL47|O_T_RL48|O_T_RL49|O_T_RL50|O_T_RH02)
      mask Display: image(imread('Output_PWM_Diagnosis.jpg'))
  Logical Operator1 : Logic  Operator=NOT  AllPortsSameDT=off  OutDataTypeStr=boolean
  Product1 : Product  OutDataTypeStr=Inherit: Same as first input
  Relational Operator : RelationalOperator  Operator===  OutDataTypeStr=boolean
  Switch1 : Switch  Threshold=1
  Switch2 : Switch  Threshold=1
  Cov_stDiagnosis : Outport
  Cov_flgError : Outport  Port=2
  wires:
  Constant6/1 -> Switch2/3
  Relational Operator/1 -> Switch2/2
  Constant5/1 -> Relational Operator/2
  Opm_idxMode/1 -> Relational Operator/1
  Switch1/1 -> Switch2/1
  dummy_facChOverVlvRate/1 -> Switch1/3
  Constant2/1 -> Switch1/1
  Constant1/1 -> Switch1/2
  Logical Operator1/1 -> Cov_flgError/1  "Cov_flgError"
  G1_PwmOut_Get_error/1(status) -> Cov_stDiagnosis/1  "Cov_stDiagnosis"
  Switch2/1 -> Product1/1  "Cov_facChOverVlvRate"
  G1_PWM_Output_Ctrl/1(status) -> Logical Operator1/1
  Constant3/1 -> Product1/2
  Product1/1 -> G1_PWM_Output_Ctrl/1(dutycycle)
  Constant7/1 -> G1_PWM_Output_Ctrl/2(period)
  Constant4/1 -> G1_PWM_Output_Ctrl/3(factor)
  Constant9/1 -> G1_PWM_Output_Ctrl/4(level)

== system M160_lib/Actuators/Fps ==
  Opm_idxMode : Inport
  dummy_stFuelPump : Inport  Port=2
  function : TriggerPort  TriggerType=function-call
  Constant1 : Constant  Value=Fps_flgFuelPumpOverride
  Constant2 : Constant  Value=Fps_stFuelPumpMan
  Constant5 : Constant  Value=Normal
  Constant6 : Constant  Value=0  OutDataTypeStr=boolean
  G1_DigOut_Ctrl : Subsystem  AncestorBlock=ehooks_medc17flex_G1_lib/Library Blocks/Basic_IO/Outputs/G1_DigOut_Ctrl  LoadFcn=ehooks_medc17flex_devlib_io_block('load');  InitFcn=ehooks_medc17flex_devlib_io_block('init');  StartFcn=ehooks_medc17flex_devlib_io_block('start');  StopFcn=ehooks_medc17flex_devlib_io_block('stop');  ClipboardFcn=ehooks_medc17flex_devlib_io_block('clipboard', 0); % Second argument just needed to indicate null block. See callback handler.  mask{ChannelName=O_S_RL09}
      mask prompts: ChannelName "Channel name"
      mask init:
      | ehooks_medc17flex_devlib_io_block('mask_init');
      settings: AttributesFormatString=Channel name: '%<ChannelName>'  CopyFcn=ehooks_medc17flex_devlib_io_block('copy');  DeleteFcn=ehooks_medc17flex_devlib_io_block('delete');  UndoDeleteFcn=ehooks_medc17flex_devlib_io_block('undo_delete');  ModelCloseFcn=ehooks_medc17flex_devlib_io_block('model_close');  PreSaveFcn=ehooks_medc17flex_devlib_io_block('pre_save');  PostSaveFcn=ehooks_medc17flex_devlib_io_block('post_save');  NameChangeFcn=ehooks_medc17flex_devlib_io_block('name_change');  DestroyFcn=ehooks_medc17flex_devlib_io_block('destroy', 0); % Second argument just needed to indicate null block. See callback handler.  OpenFcn=ehooks_medc17flex_devlib_io_block('open');  CloseFcn=ehooks_medc17flex_devlib_io_block('close');  ParentCloseFcn=ehooks_medc17flex_devlib_io_block('parent_close');  MoveFcn=ehooks_medc17flex_devlib_io_block('move');
      mask StyleString: popup(<empty>|O_S_MRLY|O_S_RL09|O_S_RL14|O_S_RL29|O_S_RL30|O_S_RL31|O_S_RL33|O_S_RL34|O_S_RL35|O_S_RL41|O_S_RL43)
      mask Display: image(imread('Output_Digital.jpg'))
  G1_DigOut_GetError : Subsystem  AncestorBlock=ehooks_medc17flex_G1_lib/Library Blocks/Basic_IO/Outputs/G1_DigOut_GetError  LoadFcn=ehooks_medc17flex_devlib_io_block('load');  InitFcn=ehooks_medc17flex_devlib_io_block('init');  StartFcn=ehooks_medc17flex_devlib_io_block('start');  StopFcn=ehooks_medc17flex_devlib_io_block('stop');  ClipboardFcn=ehooks_medc17flex_devlib_io_block('clipboard', 0); % Second argument just needed to indicate null block. See callback handler.  mask{ChannelName=O_S_RL09}
      mask prompts: ChannelName "Channel name"
      mask init:
      | ehooks_medc17flex_devlib_io_block('mask_init');
      settings: AttributesFormatString=Channel name: '%<ChannelName>'  CopyFcn=ehooks_medc17flex_devlib_io_block('copy');  DeleteFcn=ehooks_medc17flex_devlib_io_block('delete');  UndoDeleteFcn=ehooks_medc17flex_devlib_io_block('undo_delete');  ModelCloseFcn=ehooks_medc17flex_devlib_io_block('model_close');  PreSaveFcn=ehooks_medc17flex_devlib_io_block('pre_save');  PostSaveFcn=ehooks_medc17flex_devlib_io_block('post_save');  NameChangeFcn=ehooks_medc17flex_devlib_io_block('name_change');  DestroyFcn=ehooks_medc17flex_devlib_io_block('destroy', 0); % Second argument just needed to indicate null block. See callback handler.  OpenFcn=ehooks_medc17flex_devlib_io_block('open');  CloseFcn=ehooks_medc17flex_devlib_io_block('close');  ParentCloseFcn=ehooks_medc17flex_devlib_io_block('parent_close');  MoveFcn=ehooks_medc17flex_devlib_io_block('move');
      mask StyleString: popup(<empty>|O_S_MRLY|O_S_RL09|O_S_RL14|O_S_RL29|O_S_RL30|O_S_RL31|O_S_RL33|O_S_RL34|O_S_RL35|O_S_RL41|O_S_RL43)
      mask Display: image(imread('Output_Digital_Diagnosis.jpg'))
  Logical Operator1 : Logic  Operator=NOT  AllPortsSameDT=off  OutDataTypeStr=boolean
  Logical Operator2 : Logic  Operator=NOT  AllPortsSameDT=off  OutDataTypeStr=boolean
  Relational Operator : RelationalOperator  Operator===  OutDataTypeStr=boolean
  Switch1 : Switch  Threshold=1
  Switch2 : Switch  Threshold=1
  Fps_stDiagnosis : Outport
  Fps_flgError : Outport  Port=2
  wires:
  G1_DigOut_Ctrl/1(status) -> Logical Operator1/1
  Logical Operator2/1 -> G1_DigOut_Ctrl/1(state)
  Switch2/1 -> Logical Operator2/1  "Fps_stFuelPump"
  G1_DigOut_GetError/1(status) -> Fps_stDiagnosis/1  "Fps_stDiagnosis"
  Logical Operator1/1 -> Fps_flgError/1  "Fps_flgError"
  Constant1/1 -> Switch1/2
  Constant2/1 -> Switch1/1
  dummy_stFuelPump/1 -> Switch1/3
  Switch1/1 -> Switch2/1
  Opm_idxMode/1 -> Relational Operator/1
  Constant5/1 -> Relational Operator/2
  Relational Operator/1 -> Switch2/2
  Constant6/1 -> Switch2/3

== system M160_lib/Actuators/Icc ==
  note: PlaceHolder
  note: PlaceHolder
  Opm_idxMode : Inport
  Iac_flgIgnCutoff : Inport  Port=2
  Iac_degIgnIdleSpeed : Inport  Port=3
  function : TriggerPort  TriggerType=function-call
  Constant1 : Constant  Value=Icc_flgIgnCutoffOverride
  Constant10 : Constant  Value=Icc_tiOffFollowUpSparks
  Constant11 : Constant  Value=Icc_nrFollowUpSparks
  Constant{6,12..15} (5 alike) : Constant  Value=0  OutMin=-72  OutMax=78  OutDataTypeStr=single
  Constant2 : Constant  Value=Icc_flgIgnCutoffMan
  Constant3 : Constant  Value=CDRV_E_OK_
  Constant4 : Constant  Value=Icc_flgIgnAngleOverride
  Constant5 : Constant  Value=Normal
  Constant7 : Constant  Value=Icc_degIgnMan
  Constant8 : Constant  Value=Icc_tiDwell
  Constant9 : Constant  Value=Icc_tiDwellFollowUpSparks
  Demux : Demux  Outputs=8
  EdgeFalling : Subsystem
      mask Description: EdgeFalling
      mask Display: image(imread('EdgeFalling.jpg'))
  EdgeRising : Subsystem
      mask Description: EdgeRising
      mask Display: image(imread('EdgeRising.jpg'))
  G1_IGN_SetParam_for_PFI : Subsystem  AncestorBlock=ehooks_medc17flex_G1_lib/Library Blocks/IGN/IGN_PFI_Specific/G1_IGN_SetParam_for_PFI  LoadFcn=ehooks_medc17flex_devlib_io_block('load');  InitFcn=ehooks_medc17flex_devlib_io_block('init');  StartFcn=ehooks_medc17flex_devlib_io_block('start');  StopFcn=ehooks_medc17flex_devlib_io_block('stop');  ClipboardFcn=ehooks_medc17flex_devlib_io_block('clipboard', 0); % Second argument just needed to indicate null block. See callback handler.  mask{handleName=IGNORED}
      mask prompts: handleName "PlaceHolder_IGNORED"
      mask init:
      | ehooks_medc17flex_devlib_io_block('mask_init');
      settings: CopyFcn=ehooks_medc17flex_devlib_io_block('copy');  DeleteFcn=ehooks_medc17flex_devlib_io_block('delete');  UndoDeleteFcn=ehooks_medc17flex_devlib_io_block('undo_delete');  ModelCloseFcn=ehooks_medc17flex_devlib_io_block('model_close');  PreSaveFcn=ehooks_medc17flex_devlib_io_block('pre_save');  PostSaveFcn=ehooks_medc17flex_devlib_io_block('post_save');  NameChangeFcn=ehooks_medc17flex_devlib_io_block('name_change');  DestroyFcn=ehooks_medc17flex_devlib_io_block('destroy', 0); % Second argument just needed to indicate null block. See callback handler.  OpenFcn=ehooks_medc17flex_devlib_io_block('open');  CloseFcn=ehooks_medc17flex_devlib_io_block('close');  ParentCloseFcn=ehooks_medc17flex_devlib_io_block('parent_close');  MoveFcn=ehooks_medc17flex_devlib_io_block('move');
      mask StyleString: popup(IGNORED)
      mask Display: image(imread('IgnClPfi.jpg'))
  IGN_FadeOut_Immediate : Subsystem  Priority=44  AncestorBlock=ehooks_medc17flex_G1_lib/Library Blocks/IGN/IGN_Fadeout/IGN_FadeOut_Immediate  LoadFcn=ehooks_medc17flex_devlib_io_block('load');  InitFcn=ehooks_medc17flex_devlib_io_block('init');  StartFcn=ehooks_medc17flex_devlib_io_block('start');  StopFcn=ehooks_medc17flex_devlib_io_block('stop');  ClipboardFcn=ehooks_medc17flex_devlib_io_block('clipboard', 0); % Second argument just needed to indicate null block. See callback handler.  mask{ChannelName=IGNORED}
      mask prompts: ChannelName "PlaceHolder_IGNORED"
      mask init:
      | ehooks_medc17flex_devlib_io_block('mask_init');
      settings: CopyFcn=ehooks_medc17flex_devlib_io_block('copy');  DeleteFcn=ehooks_medc17flex_devlib_io_block('delete');  UndoDeleteFcn=ehooks_medc17flex_devlib_io_block('undo_delete');  ModelCloseFcn=ehooks_medc17flex_devlib_io_block('model_close');  PreSaveFcn=ehooks_medc17flex_devlib_io_block('pre_save');  PostSaveFcn=ehooks_medc17flex_devlib_io_block('post_save');  NameChangeFcn=ehooks_medc17flex_devlib_io_block('name_change');  DestroyFcn=ehooks_medc17flex_devlib_io_block('destroy', 0); % Second argument just needed to indicate null block. See callback handler.  OpenFcn=ehooks_medc17flex_devlib_io_block('open');  CloseFcn=ehooks_medc17flex_devlib_io_block('close');  ParentCloseFcn=ehooks_medc17flex_devlib_io_block('parent_close');  MoveFcn=ehooks_medc17flex_devlib_io_block('move');
      mask StyleString: popup(IGNORED)
  Logical Operator3 : Logic  Operator=OR  AllPortsSameDT=off  OutDataTypeStr=boolean
  Relational Operator : RelationalOperator  Operator=~=  OutDataTypeStr=boolean
  Relational Operator1 : RelationalOperator  Operator=~=  OutDataTypeStr=boolean
  Switch1 : Switch  Threshold=1
  Switch2 : Switch  Threshold=1
  Vector Concatenate : Concatenate  NumInputs=8  Mode=Vector
  fadeIn : Terminator
  fadeOut : Terminator
  Icc_flgError : Outport
  wires:
  Constant1/1 -> Switch1/2
  Constant2/1 -> Switch1/1
  Iac_flgIgnCutoff/1 -> Switch1/3
  Opm_idxMode/1 -> Relational Operator/1
  Constant5/1 -> Relational Operator/2
  G1_IGN_SetParam_for_PFI/1(status) -> Relational Operator1/1  "Icc_idxPfiCdrvInterfaceError"
  Relational Operator1/1 -> Icc_flgError/1  "Icc_flgError"
  Constant3/1 -> Relational Operator1/2
  Iac_degIgnIdleSpeed/1 -> Switch2/3
  Constant4/1 -> Switch2/2
  Constant7/1 -> Switch2/1
  Relational Operator/1 -> Logical Operator3/1
  Switch1/1 -> Logical Operator3/2
  Constant8/1 -> G1_IGN_SetParam_for_PFI/1(szout_w)
  Constant9/1 -> G1_IGN_SetParam_for_PFI/2(szfuba_w)
  Constant10/1 -> G1_IGN_SetParam_for_PFI/3(offz_w)
  Constant11/1 -> G1_IGN_SetParam_for_PFI/12(IGN_fubaanz)
  Logical Operator3/1 -> EdgeRising/1(signal), EdgeFalling/1(signal)  "Icc_stIgnFadeOutReq"
  Demux/1 -> G1_IGN_SetParam_for_PFI/4(IGN_zwcalcar_1)
  Demux/2 -> G1_IGN_SetParam_for_PFI/5(IGN_zwcalcar_2)
  Demux/3 -> G1_IGN_SetParam_for_PFI/6(IGN_zwcalcar_3)
  Demux/4 -> G1_IGN_SetParam_for_PFI/7(IGN_zwcalcar_4)
  Demux/5 -> G1_IGN_SetParam_for_PFI/8(IGN_zwcalcar_5)
  Demux/6 -> G1_IGN_SetParam_for_PFI/9(IGN_zwcalcar_6)
  Demux/7 -> G1_IGN_SetParam_for_PFI/10(IGN_zwcalcar_7)
  Demux/8 -> G1_IGN_SetParam_for_PFI/11(IGN_zwcalcar_8)
  Vector Concatenate/1 -> Demux/1  "Icc_degIgn_Arr"
  Constant6/1 -> Vector Concatenate/4
  Constant12/1 -> Vector Concatenate/5
  Constant13/1 -> Vector Concatenate/6
  Constant14/1 -> Vector Concatenate/7
  Constant15/1 -> Vector Concatenate/8
  Switch2/1 -> Vector Concatenate/2, Vector Concatenate/1, Vector Concatenate/3
  EdgeFalling/1(return) -> fadeIn/1
  EdgeRising/1(return) -> fadeOut/1

== system M160_lib/Actuators/Ics ==
  Opm_idxMode : Inport
  dummy_stIntercooler : Inport  Port=2
  function : TriggerPort  TriggerType=function-call
  Constant1 : Constant  Value=Ics_flgIntercoolerOverride
  Constant2 : Constant  Value=Ics_stIntercoolerMan
  Constant5 : Constant  Value=Normal
  Constant6 : Constant  Value=0  OutDataTypeStr=boolean
  G1_DigOut_Ctrl : Subsystem  AncestorBlock=ehooks_medc17flex_G1_lib/Library Blocks/Basic_IO/Outputs/G1_DigOut_Ctrl  LoadFcn=ehooks_medc17flex_devlib_io_block('load');  InitFcn=ehooks_medc17flex_devlib_io_block('init');  StartFcn=ehooks_medc17flex_devlib_io_block('start');  StopFcn=ehooks_medc17flex_devlib_io_block('stop');  ClipboardFcn=ehooks_medc17flex_devlib_io_block('clipboard', 0); % Second argument just needed to indicate null block. See callback handler.  mask{ChannelName=O_S_RL29}
      mask prompts: ChannelName "Channel name"
      mask init:
      | ehooks_medc17flex_devlib_io_block('mask_init');
      settings: AttributesFormatString=Channel name: '%<ChannelName>'  CopyFcn=ehooks_medc17flex_devlib_io_block('copy');  DeleteFcn=ehooks_medc17flex_devlib_io_block('delete');  UndoDeleteFcn=ehooks_medc17flex_devlib_io_block('undo_delete');  ModelCloseFcn=ehooks_medc17flex_devlib_io_block('model_close');  PreSaveFcn=ehooks_medc17flex_devlib_io_block('pre_save');  PostSaveFcn=ehooks_medc17flex_devlib_io_block('post_save');  NameChangeFcn=ehooks_medc17flex_devlib_io_block('name_change');  DestroyFcn=ehooks_medc17flex_devlib_io_block('destroy', 0); % Second argument just needed to indicate null block. See callback handler.  OpenFcn=ehooks_medc17flex_devlib_io_block('open');  CloseFcn=ehooks_medc17flex_devlib_io_block('close');  ParentCloseFcn=ehooks_medc17flex_devlib_io_block('parent_close');  MoveFcn=ehooks_medc17flex_devlib_io_block('move');
      mask StyleString: popup(<empty>|O_S_MRLY|O_S_RL09|O_S_RL14|O_S_RL29|O_S_RL30|O_S_RL31|O_S_RL33|O_S_RL34|O_S_RL35|O_S_RL41|O_S_RL43)
      mask Display: image(imread('Output_Digital.jpg'))
  G1_DigOut_GetError : Subsystem  AncestorBlock=ehooks_medc17flex_G1_lib/Library Blocks/Basic_IO/Outputs/G1_DigOut_GetError  LoadFcn=ehooks_medc17flex_devlib_io_block('load');  InitFcn=ehooks_medc17flex_devlib_io_block('init');  StartFcn=ehooks_medc17flex_devlib_io_block('start');  StopFcn=ehooks_medc17flex_devlib_io_block('stop');  ClipboardFcn=ehooks_medc17flex_devlib_io_block('clipboard', 0); % Second argument just needed to indicate null block. See callback handler.  mask{ChannelName=O_S_RL29}
      mask prompts: ChannelName "Channel name"
      mask init:
      | ehooks_medc17flex_devlib_io_block('mask_init');
      settings: AttributesFormatString=Channel name: '%<ChannelName>'  CopyFcn=ehooks_medc17flex_devlib_io_block('copy');  DeleteFcn=ehooks_medc17flex_devlib_io_block('delete');  UndoDeleteFcn=ehooks_medc17flex_devlib_io_block('undo_delete');  ModelCloseFcn=ehooks_medc17flex_devlib_io_block('model_close');  PreSaveFcn=ehooks_medc17flex_devlib_io_block('pre_save');  PostSaveFcn=ehooks_medc17flex_devlib_io_block('post_save');  NameChangeFcn=ehooks_medc17flex_devlib_io_block('name_change');  DestroyFcn=ehooks_medc17flex_devlib_io_block('destroy', 0); % Second argument just needed to indicate null block. See callback handler.  OpenFcn=ehooks_medc17flex_devlib_io_block('open');  CloseFcn=ehooks_medc17flex_devlib_io_block('close');  ParentCloseFcn=ehooks_medc17flex_devlib_io_block('parent_close');  MoveFcn=ehooks_medc17flex_devlib_io_block('move');
      mask StyleString: popup(<empty>|O_S_MRLY|O_S_RL09|O_S_RL14|O_S_RL29|O_S_RL30|O_S_RL31|O_S_RL33|O_S_RL34|O_S_RL35|O_S_RL41|O_S_RL43)
      mask Display: image(imread('Output_Digital_Diagnosis.jpg'))
  Logical Operator1 : Logic  Operator=NOT  AllPortsSameDT=off  OutDataTypeStr=boolean
  Logical Operator2 : Logic  Operator=NOT  AllPortsSameDT=off  OutDataTypeStr=boolean
  Relational Operator : RelationalOperator  Operator===  OutDataTypeStr=boolean
  Switch1 : Switch  Threshold=1
  Switch2 : Switch  Threshold=1
  Ics_stDiagnosis : Outport
  Ics_flgError : Outport  Port=2
  wires:
  Constant6/1 -> Switch2/3
  Relational Operator/1 -> Switch2/2
  Constant5/1 -> Relational Operator/2
  Opm_idxMode/1 -> Relational Operator/1
  Switch1/1 -> Switch2/1
  dummy_stIntercooler/1 -> Switch1/3
  Constant2/1 -> Switch1/1
  Constant1/1 -> Switch1/2
  Logical Operator1/1 -> Ics_flgError/1  "Ics_flgError"
  G1_DigOut_GetError/1(status) -> Ics_stDiagnosis/1  "Ics_stDiagnosis"
  Switch2/1 -> Logical Operator2/1  "Ics_stIntercooler"
  Logical Operator2/1 -> G1_DigOut_Ctrl/1(state)
  G1_DigOut_Ctrl/1(status) -> Logical Operator1/1
